simulink model "tyre"  (R2025b)
settings: Solver=VariableStepAuto  StartTime=0.0  StopTime=simin.Time.data(end)  RelTol=1e-3
model workspace (MAT data in the model file):
  F_z0 = Simulink.Parameter
  F_z0.Value = 6500
  F_z0.Complexity = 'real'
  F_z0.Dimensions = [1 1]
  F_z0.DataType = 'double'
  F_z0.DocUnits = 'N'
  Fz_stat_FL = Simulink.Parameter
  Fz_stat_FL.Value = 3921.3656
  Fz_stat_FL.Complexity = 'real'
  Fz_stat_FL.Dimensions = [1 1]
  Fz_stat_FL.DataType = 'double'
  Fz_stat_FL.DocUnits = 'N'
  Fz_stat_FR = Simulink.Parameter
  Fz_stat_FR.Value = 3921.3656
  Fz_stat_FR.Complexity = 'real'
  Fz_stat_FR.Dimensions = [1 1]
  Fz_stat_FR.DataType = 'double'
  Fz_stat_FR.DocUnits = 'N'
  Fz_stat_RL = Simulink.Parameter
  Fz_stat_RL.Value = 3922.1269
  Fz_stat_RL.Complexity = 'real'
  Fz_stat_RL.Dimensions = [1 1]
  Fz_stat_RL.DataType = 'double'
  Fz_stat_RL.DocUnits = 'N'
  Fz_stat_RR = Simulink.Parameter
  Fz_stat_RR.Value = 3922.1267
  Fz_stat_RR.Complexity = 'real'
  Fz_stat_RR.Dimensions = [1 1]
  Fz_stat_RR.DataType = 'double'
  Fz_stat_RR.DocUnits = 'N'
  c_z = Simulink.Parameter
  c_z.Value = 236700
  c_z.Complexity = 'real'
  c_z.Dimensions = [1 1]
  c_z.DataType = 'double'
  c_z.DocUnits = 'N/m'
  cog_height = Simulink.Parameter
  cog_height.Value = 0.604
  cog_height.Complexity = 'real'
  cog_height.Dimensions = [1 1]
  cog_height.DataType = 'double'
  cog_height.DocUnits = 'm'
  d_reff = Simulink.Parameter
  d_reff.Value = 0.3
  d_reff.Complexity = 'real'
  d_reff.Dimensions = [1 1]
  d_reff.DataType = 'double'
  d_reff.DocUnits = 'm'
  f_reff = Simulink.Parameter
  f_reff.Value = 0.1
  f_reff.Complexity = 'real'
  f_reff.Dimensions = [1 1]
  f_reff.DataType = 'double'
  f_reff.DocUnits = 'N/m'
  g = Simulink.Parameter
  g.Value = 9.806
  g.Complexity = 'real'
  g.Dimensions = [1 1]
  g.DataType = 'double'
  g.DocUnits = 'm/s^2'
  lF = Simulink.Parameter
  lF.Value = 1.466
  lF.Complexity = 'real'
  lF.Dimensions = [1 1]
  lF.DataType = 'double'
  lF.DocUnits = 'm'
  lR = Simulink.Parameter
  lR.Value = 1.509
  lR.Complexity = 'real'
  lR.Dimensions = [1 1]
  lR.DataType = 'double'
  lR.DocUnits = 'm'
  pitchAngle = Simulink.Parameter
  pitchAngle.Value = [0.00443372596055 0.00472012698538 0.00500652801021 0.00529292903504 0.00557933005986 0.00586573108469 0.00615213210952 0.00643853313435 0.00672493415917 0.007011335184 0.00729773620883 0.00758413723366 ... (200 elements, 200x1)]
  pitchAngle.Complexity = 'real'
  pitchAngle.Dimensions = [200 1]
  pitchAngle.DataType = 'double'
  pitchAngle.DocUnits = 'rad'
  pitchStiffness = Simulink.Parameter
  pitchStiffness.Value = [286621.759635 286644.842257 286407.773968 286374.136656 286600.567598 286901.705993 287109.32323 287190.659823 287245.018359 287344.728913 287488.533524 287631.863692 ... (200 elements, 200x1)]
  pitchStiffness.Complexity = 'real'
  pitchStiffness.Dimensions = [200 1]
  pitchStiffness.DataType = 'double'
  pitchStiffness.DocUnits = 'N*m/rad'
  pitch_inertia = Simulink.Parameter
  pitch_inertia.Value = 2180.5
  pitch_inertia.Complexity = 'real'
  pitch_inertia.Dimensions = [1 1]
  pitch_inertia.DataType = 'double'
  pitch_inertia.DocUnits = 'kg * m^2'
  pitching_coefficient = Simulink.Parameter
  pitching_coefficient.Value = -0.002
  pitching_coefficient.Complexity = 'real'
  pitching_coefficient.Dimensions = [1 1]
  pitching_coefficient.DataType = 'double'
  pitching_coefficient.DocUnits = '1'
  r_0 = Simulink.Parameter
  r_0.Value = 0.3185
  r_0.Complexity = 'real'
  r_0.Dimensions = [1 1]
  r_0.DataType = 'double'
  r_0.DocUnits = 'm'
  rdyn = Simulink.Parameter
  rdyn.Value = 0.309
  rdyn.Complexity = 'real'
  rdyn.Dimensions = [1 1]
  rdyn.DataType = 'double'
  rdyn.DocUnits = 'm'
  reference_area = Simulink.Parameter
  reference_area.Value = 2.4
  reference_area.Complexity = 'real'
  reference_area.Dimensions = [1 1]
  reference_area.DataType = 'double'
  reference_area.DocUnits = 'kg / m^3'
  rho = Simulink.Parameter
  rho.Value = 1.2
  rho.Complexity = 'real'
  rho.Dimensions = [1 1]
  rho.DataType = 'double'
  rho.DocUnits = 'm^2'
  rollStiffness_F = Simulink.Parameter
  rollStiffness_F.Value = -66168.4036
  rollStiffness_F.Complexity = 'real'
  rollStiffness_F.Dimensions = [1 1]
  rollStiffness_F.DataType = 'double'
  rollStiffness_F.DocUnits = 'N*m/rad'
  rollStiffness_R = Simulink.Parameter
  rollStiffness_R.Value = -79058.3706
  rollStiffness_R.Complexity = 'real'
  rollStiffness_R.Dimensions = [1 1]
  rollStiffness_R.DataType = 'double'
  rollStiffness_R.DocUnits = 'N*m/rad'
  sprung_mass = Simulink.Parameter
  sprung_mass.Value = 1373.3
  sprung_mass.Complexity = 'real'
  sprung_mass.Dimensions = [1 1]
  sprung_mass.DataType = 'double'
  sprung_mass.DocUnits = 'kg'
  tire = Simulink.Parameter
  tire.Value.MDI_Header.FILE_VERSION = 2
  tire.Value.Model.USE_MODE = 14
  tire.Value.Dim.UNLOADED_RADIUS = 0.3185
  tire.Value.Dim.WIDTH = 0.205
  tire.Value.Dim.RIM_RADIUS = 0.1905
  tire.Value.Dim.RIM_WIDTH = 0.1524
  tire.Value.Dim.ASPECT_RATIO = 0.6
  tire.Value.Vertical.VERTICAL_STIFFNESS = 236700
  tire.Value.Vertical.VERTICAL_DAMPING = 50
  tire.Value.Vertical.BREFF = 5
  tire.Value.Vertical.DREFF = 0.3
  tire.Value.Vertical.FREFF = 0.1
  tire.Value.Vertical.FNOMIN = 6500
  tire.Value.Range.KPUMIN = -0.3
  tire.Value.Range.KPUMAX = 0.3
  tire.Value.Range.ALPMIN = -0.1745
  tire.Value.Range.ALPMAX = 0.1745
  tire.Value.Range.CAMMIN = -0.1047
  tire.Value.Range.CAMMAX = 0.1047
  tire.Value.Range.FZMIN = 400
  tire.Value.Range.FZMAX = 8500
  tire.Value.Scale.LFZO = 1
  tire.Value.Scale.LCX = 1
  tire.Value.Scale.LMUX = 1
  tire.Value.Scale.LEX = 1
  tire.Value.Scale.LKX = 1
  tire.Value.Scale.LHX = 1
  tire.Value.Scale.LVX = 1
  tire.Value.Scale.LGAX = 1
  tire.Value.Scale.LCY = 1
  tire.Value.Scale.LMUY = 1
  tire.Value.Scale.LEY = 1
  tire.Value.Scale.LKY = 1
  tire.Value.Scale.LHY = 1
  tire.Value.Scale.LVY = 1
  tire.Value.Scale.LGAY = 1
  tire.Value.Scale.LTR = 1
  tire.Value.Scale.LRES = 1
  tire.Value.Scale.LGAZ = 1
  tire.Value.Scale.LXAL = 1
  tire.Value.Scale.LYKA = 1
  tire.Value.Scale.LVYKA = 1
  tire.Value.Scale.LS = 1
  tire.Value.Scale.LSGKP = 1
  tire.Value.Scale.LSGAL = 1
  tire.Value.Scale.LGYR = 1
  tire.Value.Scale.LMX = 1
  tire.Value.Scale.LVMX = 1
  tire.Value.Scale.LMY = 1
  tire.Value.Long.PCX1 = 1.6055
  tire.Value.Long.PDX1 = 1.1703
  tire.Value.Long.PDX2 = -0.081328
  tire.Value.Long.PDX3 = 0
  tire.Value.Long.PEX1 = 0.53409
  tire.Value.Long.PEX2 = -0.019956
  tire.Value.Long.PEX3 = 0.18089
  tire.Value.Long.PEX4 = 2.9951e-07
  tire.Value.Long.PKX1 = 36.411
  tire.Value.Long.PKX2 = 0.12615
  tire.Value.Long.PKX3 = 0.51289
  tire.Value.Long.PHX1 = 0
  tire.Value.Long.PHX2 = 0
  tire.Value.Long.PVX1 = 0
  tire.Value.Long.PVX2 = 0
  tire.Value.Long.RBX1 = 18.456
  tire.Value.Long.RBX2 = 16.314
  tire.Value.Long.RCX1 = 1.091
  tire.Value.Long.REX1 = 0
  tire.Value.Long.REX2 = 0
  tire.Value.Long.RHX1 = 0.0058715
  tire.Value.Long.PTX1 = 1.5
  tire.Value.Long.PTX2 = 0.180096
  tire.Value.Long.PTX3 = -0.15
  tire.Value.OverTurn.QSX1 = 0.00023155
  tire.Value.OverTurn.QSX2 = 0.51574
  tire.Value.OverTurn.QSX3 = 0.046399
  tire.Value.Lat.PCY1 = 2.1322
  tire.Value.Lat.PDY1 = 1.0283
  tire.Value.Lat.PDY2 = -0.16758
  tire.Value.Lat.PDY3 = -1.5821
  tire.Value.Lat.PEY1 = 0.33443
  tire.Value.Lat.PEY2 = -1.8733
  tire.Value.Lat.PEY3 = -0.13136
  tire.Value.Lat.PEY4 = -11.677
  tire.Value.Lat.PKY1 = -20.505
  tire.Value.Lat.PKY2 = 2.0284
  tire.Value.Lat.PKY3 = 0.89994
  tire.Value.Lat.PHY1 = 0.0031377
  tire.Value.Lat.PHY2 = 0.00051596
  tire.Value.Lat.PHY3 = 0.039251
  tire.Value.Lat.PVY1 = 0.026365
  tire.Value.Lat.PVY2 = -0.0062119
  tire.Value.Lat.PVY3 = -0.41389
  tire.Value.Lat.PVY4 = -0.048038
  tire.Value.Lat.RBY1 = 22.003
  tire.Value.Lat.RBY2 = -13.623
  tire.Value.Lat.RBY3 = -0.0093616
  tire.Value.Lat.RCY1 = 0.98294
  tire.Value.Lat.REY1 = 0
  tire.Value.Lat.REY2 = 0
  tire.Value.Lat.RHY1 = -9.1492e-11
  tire.Value.Lat.RHY2 = 0
  tire.Value.Lat.RVY1 = 22.965
  tire.Value.Lat.RVY2 = 0.37981
  tire.Value.Lat.RVY3 = 1.8552
  tire.Value.Lat.RVY4 = 0.08767
  tire.Value.Lat.RVY5 = -8.8234e-11
  tire.Value.Lat.RVY6 = 0.90374
  tire.Value.Lat.PTY1 = 1.75
  tire.Value.Lat.PTY2 = 1.35
  tire.Value.Roll.QSY1 = 0.01
  tire.Value.Roll.QSY2 = 0
  tire.Value.Roll.QSY3 = 0
  tire.Value.Roll.QSY4 = 0
  tire.Value.Align.QBZ1 = 19.588
  tire.Value.Align.QBZ2 = -4.1671
  tire.Value.Align.QBZ3 = -0.34132
  tire.Value.Align.QBZ4 = -0.023607
  tire.Value.Align.QBZ5 = -0.0793
  tire.Value.Align.QBZ9 = -50
  tire.Value.Align.QBZ10 = 0
  tire.Value.Align.QCZ1 = 1.2012
  tire.Value.Align.QDZ1 = 0.12819
  tire.Value.Align.QDZ2 = -0.0052433
  tire.Value.Align.QDZ3 = -0.099544
  tire.Value.Align.QDZ4 = -15
  tire.Value.Align.QDZ6 = 6.2499e-05
  tire.Value.Align.QDZ7 = 0.00050135
  tire.Value.Align.QDZ8 = -0.28564
  tire.Value.Align.QDZ9 = -0.025056
  tire.Value.Align.QEZ1 = -0.0044308
  tire.Value.Align.QEZ2 = 0.022579
  tire.Value.Align.QEZ3 = -0.16199
  tire.Value.Align.QEZ4 = -0.5576
  tire.Value.Align.QEZ5 = -87.296
  tire.Value.Align.QHZ1 = 0.00082436
  tire.Value.Align.QHZ2 = 0.002733
  tire.Value.Align.QHZ3 = 0.15
  tire.Value.Align.QHZ4 = 0.11608
  tire.Value.Align.SSZ1 = -5.3899e-10
  tire.Value.Align.SSZ2 = -2.2371e-09
  tire.Value.Align.SSZ3 = 3.6029e-08
  tire.Value.Align.SSZ4 = 3.9826e-08
  tire.Value.Align.QTZ1 = 0.3
  tire.Value.Align.MBELT = 7.5
  tire.Value.FLoadMax = 10000
  tire.Complexity = 'real'
  tire.Dimensions = [1 1]
  tire.DataType = 'struct'
  total_pitchDamping = Simulink.Parameter
  total_pitchDamping.Value = 22000
  total_pitchDamping.Complexity = 'real'
  total_pitchDamping.Dimensions = [1 1]
  total_pitchDamping.DataType = 'double'
  total_pitchDamping.DocUnits = 'N*m/rad'
  total_pitchStiffness = Simulink.Parameter
  total_pitchStiffness.Value = 291158.1055
  total_pitchStiffness.Complexity = 'real'
  total_pitchStiffness.Dimensions = [1 1]
  total_pitchStiffness.DataType = 'double'
  total_pitchStiffness.DocUnits = 'N*m/rad'
  total_rollStiffness = Simulink.Parameter
  total_rollStiffness.Value = 138201.9734
  total_rollStiffness.Complexity = 'real'
  total_rollStiffness.Dimensions = [1 1]
  total_rollStiffness.DataType = 'double'
  total_rollStiffness.DocUnits = 'N*m/rad'
  trackwidth_F = Simulink.Parameter
  trackwidth_F.Value = 1.6
  trackwidth_F.Complexity = 'real'
  trackwidth_F.Dimensions = [1 1]
  trackwidth_F.DataType = 'double'
  trackwidth_F.DocUnits = 'm'
  trackwidth_R = Simulink.Parameter
  trackwidth_R.Value = 1.614
  trackwidth_R.Complexity = 'real'
  trackwidth_R.Dimensions = [1 1]
  trackwidth_R.DataType = 'double'
  trackwidth_R.DocUnits = 'm'
  unsprung_mass = Simulink.Parameter
  unsprung_mass.Value = 226.704
  unsprung_mass.Complexity = 'real'
  unsprung_mass.Dimensions = [1 1]
  unsprung_mass.DataType = 'double'
  unsprung_mass.DocUnits = 'kg'
  wheelbase = Simulink.Parameter
  wheelbase.Value = 2.975
  wheelbase.Complexity = 'real'
  wheelbase.Dimensions = [1 1]
  wheelbase.DataType = 'double'
  wheelbase.DocUnits = 'm'
undefined symbols (not defined in the file): b_reff, track_width_F, track_width_R
settings Model: Creator=marcelkaminski  LastModifiedBy=marce

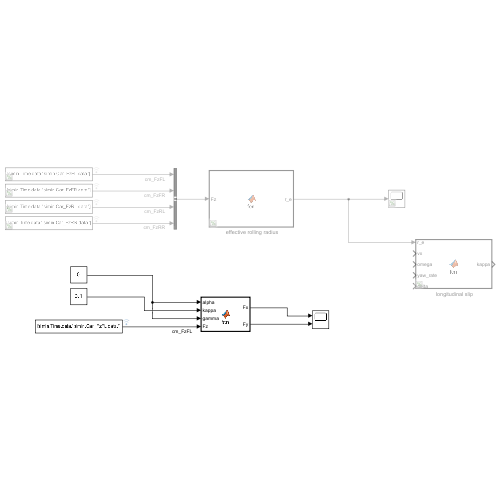
[thumbnail: Simulink's stored preview of the top-level diagram]
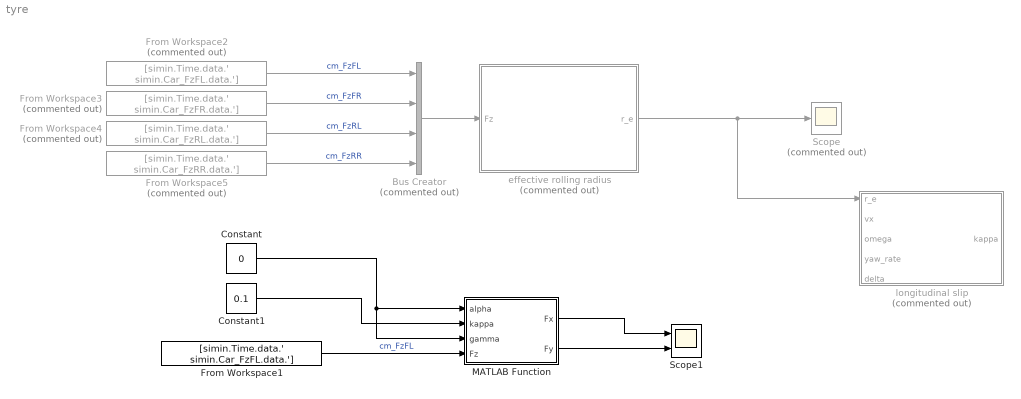
== system tyre ==
  " effective rolling radius" : MATLAB Function  Commented=on  TreatAsAtomicUnit=on
  " longitudinal slip" : MATLAB Function  Commented=on  TreatAsAtomicUnit=on
  Bus Creator : BusCreator  Commented=on  Inputs=4
  Constant : Constant  Value=0
  Constant1 : Constant  Value=0.1
  From Workspace1 : FromWorkspace  VariableName=[simin.Time.data.' simin.Car_FzFL.data.']  SampleTime=0.01
  From Workspace2 : FromWorkspace  Commented=on  VariableName=[simin.Time.data.' simin.Car_FzFL.data.']  SampleTime=0.01
  From Workspace3 : FromWorkspace  Commented=on  VariableName=[simin.Time.data.' simin.Car_FzFR.data.']  SampleTime=0.01
  From Workspace4 : FromWorkspace  Commented=on  VariableName=[simin.Time.data.' simin.Car_FzRL.data.']  SampleTime=0.01
  From Workspace5 : FromWorkspace  Commented=on  VariableName=[simin.Time.data.' simin.Car_FzRR.data.']  SampleTime=0.01
  MATLAB Function : MATLAB Function  TreatAsAtomicUnit=on
  Scope : Scope  Commented=on
      settings: ActiveDisplayYMinimum=0.30410339136461506  ActiveDisplayYMaximum=0.30918504692485255
  Scope1 : Scope  NumInputPorts=2
      settings: ActiveDisplayYMinimum=-662.77029509835268  ActiveDisplayYMaximum=5297.5716410991763
  wires:
  From Workspace5/1 -> Bus Creator/4  "cm_FzRR"
  From Workspace3/1 -> Bus Creator/2  "cm_FzFR"
  From Workspace2/1 -> Bus Creator/1  "cm_FzFL"
  From Workspace4/1 -> Bus Creator/3  "cm_FzRL"
  Bus Creator/1 -> " effective rolling radius"/1(Fz)
  " effective rolling radius"/1(r_e) -> " longitudinal slip"/1(r_e), Scope/1
  MATLAB Function/1(Fx) -> Scope1/1
  From Workspace1/1 -> MATLAB Function/4(Fz)  "cm_FzFL"
  Constant/1 -> MATLAB Function/3(gamma), MATLAB Function/1(alpha)
  Constant1/1 -> MATLAB Function/2(kappa)
  MATLAB Function/2(Fy) -> Scope1/2

== matlab function tyre/ longitudinal slip ==
  data: r_e input; vx input; kappa output; omega input; yaw_rate input; delta input; track_width_F parameter; track_width_R parameter
function kappa = fcn(r_e,vx,omega,yaw_rate,delta,track_width_F, track_width_R)

    vx_lon_FL = (vx + yaw_rate * 0.5 * track_width_F) / cos(delta(1));
    vx_lon_FR = (vx - yaw_rate * 0.5 * track_width_F) / cos(delta(2));
    vx_lon_RL = (vx + yaw_rate * 0.5 * track_width_R) / cos(delta(3));
    vx_lon_RR = (vx - yaw_rate * 0.5 * track_width_R) / cos(delta(3));
    
    v_sx_FL = vx_lon_FL - (omega(1)*r_e(1));
    v_sx_FR = vx_lon_FR - (omega(2)*r_e(2));
    v_sx_RL = vx_lon_RL - (omega(3)*r_e(3));
    v_sx_RR = vx_lon_RR - (omega(4)*r_e(4));
    
    kappa_FL = -(v_sx_FL/vx_lon_FL);
    kappa_FR = -(v_sx_FR/vx_lon_FR);
    kappa_RL = -(v_sx_RL/vx_lon_RL);
    kappa_RR = -(v_sx_RR/vx_lon_RR);
    
    kappa = [kappa_FL,kappa_FR,kappa_RL,kappa_RR];

== matlab function tyre/ effective rolling radius ==
  data: Fz input; r_e output; c_z parameter; b_reff parameter; d_reff parameter; f_reff parameter; F_z0 parameter; r_0 parameter
function r_e  = fcn(Fz,c_z, b_reff, d_reff, f_reff, F_z0, r_0)

    p_FL = Fz(1) / c_z;
    p_FR = Fz(2) / c_z;
    p_RL = Fz(3) / c_z;
    p_RR = Fz(4) / c_z;

    p_Fz0 = F_z0 / c_z;

    p_d_FL = p_FL / p_Fz0;
    p_d_FR = p_FR / p_Fz0;
    p_d_RL = p_RL / p_Fz0;
    p_d_RR = p_RR / p_Fz0;

    r_e_FL = r_0 - (p_Fz0 * (d_reff * atan(b_reff * p_d_FL) + f_reff * p_d_FL));
    r_e_FR = r_0 - (p_Fz0 * (d_reff * atan(b_reff * p_d_FR) + f_reff * p_d_FR));
    r_e_RL = r_0 - (p_Fz0 * (d_reff * atan(b_reff * p_d_RL) + f_reff * p_d_RL));
    r_e_RR = r_0 - (p_Fz0 * (d_reff * atan(b_reff * p_d_RR) + f_reff * p_d_RR));

    r_e = [r_e_FL, r_e_FR, r_e_RL, r_e_RR];

== matlab function tyre/MATLAB Function ==
  data: alpha input; kappa input; gamma input; Fz input; Fx output; tire parameter; Fy output
function [Fx, Fy]= fcn(alpha, kappa, gamma, Fz, tire)
    %% parameter
    
    % general
    Fz0 = tire.Vertical.FNOMIN;
    
    % longitudinal (pure slip)
    p_Cx1 = tire.Long.PCX1;
    
    p_Dx1 = tire.Long.PDX1;
    p_Dx2 = tire.Long.PDX2;
    p_Dx3 = tire.Long.PDX3;
    
    p_Ex1 = tire.Long.PEX1;
    p_Ex2 = tire.Long.PEX2;
    p_Ex3 = tire.Long.PEX3;
    p_Ex4 = tire.Long.PEX4;
    
    p_Kx1 = tire.Long.PKX1;
    p_Kx2 = tire.Long.PKX2;
    p_Kx3 = tire.Long.PKX3;
    
    p_Hx1 = tire.Long.PHX1;
    p_Hx2 = tire.Long.PHX2;
    
    p_Vx1 = tire.Long.PVX1;
    p_Vx2 = tire.Long.PVX2;
    
    % lateral (pure slip)
    p_Cy1 = tire.Lat.PCY1;
    
    p_Dy1 = tire.Lat.PDY1;
    p_Dy2 = tire.Lat.PDY2;
    p_Dy3 = tire.Lat.PDY3;
    
    p_Ey1 = tire.Lat.PEY1;
    p_Ey2 = tire.Lat.PEY2;
    p_Ey3 = tire.Lat.PEY3;
    p_Ey4 = tire.Lat.PEY4;
    
    p_Ky1 = tire.Lat.PKY1;
    p_Ky2 = tire.Lat.PKY2;
    p_Ky3 = tire.Lat.PKY3;
    
    p_Hy1 = tire.Lat.PHY1;
    p_Hy2 = tire.Lat.PHY2;
    p_Hy3 = tire.Lat.PHY3;
    
    p_Vy1 = tire.Lat.PVY1;
    p_Vy2 = tire.Lat.PVY2;
    p_Vy3 = tire.Lat.PVY3;
    p_Vy4 = tire.Lat.PVY4;
    
    % longitudinal (combined slip)
    r_Bx1 = tire.Long.RBX1;
    r_Bx2 = tire.Long.RBX2;
    
    r_Cx1 = tire.Long.RCX1;
    
    r_Ex1 = tire.Long.REX1;
    r_Ex2 = tire.Long.REX2;
    
    r_Hx1 = tire.Long.RHX1;
    
    % lateral (combined slip)
    r_By1 = tire.Lat.RBY1;
    r_By2 = tire.Lat.RBY2;
    r_By3 = tire.Lat.RBY3;
    
    r_Cy1 = tire.Lat.RCY1;
    
    r_Ey1 = tire.Lat.REY1;
    r_Ey2 = tire.Lat.REY2;
    
    r_Hy1 = tire.Lat.RHY1;
    r_Hy2 = tire.Lat.RHY2;
    
    r_Vy1 = tire.Lat.RVY1;
    r_Vy2 = tire.Lat.RVY2;
    r_Vy3 = tire.Lat.RVY3;
    r_Vy4 = tire.Lat.RVY4;
    r_Vy5 = tire.Lat.RVY5;
    r_Vy6 = tire.Lat.RVY6;
    
    %% calculations
    
    % general
    dfz = ((Fz-Fz0)/Fz0);
    
    % longitudinal (pure slip)
    Cx = p_Cx1;
    
    mu_x = (p_Dx1 + p_Dx2 .* dfz) .* (1 - p_Dx3 .* gamma.^2);
    Dx = mu_x .* Fz;
    
    S_Hx = (p_Hx1 + p_Hx2 .* dfz);
    S_Vx = Fz .* (p_Vx1 + p_Vx2 .* dfz);
    
    kappa_x = kappa + S_Hx;
    
    Ex = (p_Ex1 + p_Ex2 .* dfz + p_Ex3 .* dfz.^2) .* (1 - p_Ex4 .* sign(kappa_x));
    Kx = Fz .* (p_Kx1 + p_Kx2 .* dfz) .* exp(p_Kx3 .* dfz);
    Bx = Kx ./ (Cx .* Dx);
    
    Fx0 = Dx .* sin(Cx .* atan(Bx .* kappa_x - Ex .* (Bx .* kappa_x - atan(Bx .* kappa_x)))) + S_Vx;
    
    % lateral (pure slip)
    Cy = p_Cy1;
    
    mu_y = (p_Dy1 + p_Dy2 .* dfz) .* (1-p_Dy3 .* gamma.^2);
    Dy = mu_y .* Fz;
    
    S_Hy = p_Hy1 + p_Hy2 + p_Hy3 .* gamma;
    S_Vy = Fz .* (p_Vy1 + p_Vy2 .* dfz + (p_Vy3 + p_Vy4 .* dfz) .* gamma);
    
    alpha_y = alpha + S_Hy;
    
    Ey = (p_Ey1 + p_Ey2 .* dfz) .* (1 - (p_Ey3 + p_Ey4 .* gamma) .* sign(alpha_y));
    Ky = p_Ky1 .* Fz0 .* sin(2 .* atan(Fz / (p_Ky2 .* Fz0))) .* (1 - p_Ky3 .* abs(gamma));
    By = Ky / (Cy .* Dy);
    
    Fy0 = Dy .* sin(Cy .* atan(By .* alpha_y - Ey .* (By .* alpha_y - atan(By .* alpha_y)))) + S_Vy;
    
    % longitudinal (combined slip)
    S_Hxa = r_Hx1;
    alpha_s = alpha + S_Hxa;
    
    Bxa = r_Bx1 .* cos(atan(r_Bx2 .* kappa));
    Cxa = r_Cx1;
    Exa = r_Ex1 + r_Ex2 .* dfz;
    
    Gxa = (cos(Cxa .* atan(Bxa .* alpha_s - Exa .* (Bxa .* alpha_s - atan(Bxa .*alpha_s))))) ./ ...
        (cos(Cxa .* atan(Bxa .* S_Hxa - Exa .* (Bxa .* S_Hxa - atan(Bxa .* S_Hxa)))));
    
    Fx = Fx0 .* Gxa;
    
    % lateral (combined slip)
    S_Hyk = r_Hy1 + r_Hy2 .* dfz;
    kappa_s = kappa + S_Hyk;
    
    Byk = r_By1 .* cos(atan(r_By2 .* (alpha-r_By3)));
    Cyk = r_Cy1;
    Eyk = r_Ey1 + r_Ey2 .* dfz;
    
    D_Vyk = mu_y .* Fz .* (r_Vy1 + r_Vy2 .* dfz + r_Vy3 .* gamma) .* cos(atan(r_Vy4 .* alpha));
    S_Vyk = D_Vyk .* sin(r_Vy5 .* atan(r_Vy6 .* kappa));
    
    Gyk = (cos(Cyk .* atan(Byk .* kappa_s - Eyk .* (Byk .* kappa_s - atan(Byk .* kappa_s))))) ./ ...
        (cos(Cyk .* atan(Byk .* S_Hyk - Eyk .* (Byk .* S_Hyk - atan(Byk .* S_Hyk)))));
    
    Fy = Fy0 .* Gyk + S_Vyk;
